simulink model "FPGA_Comm_test_plant"  (Simulink 7.6)
settings: Solver=ode4  StartTime=0.0  StopTime=500  FixedStep=0.01  MaxStep=1e-1  RelTol=1e-3
values from neighbouring files (symbols this model uses):
  s1 = op1(1)    [fpu_test.m]
settings Model: Creator=jordan  LastModifiedBy=jordan
settings GRTTargetCC: ExtMode=on

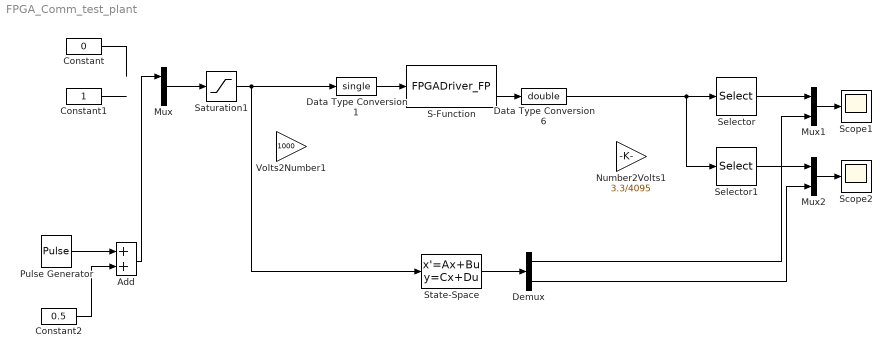
== system FPGA_Comm_test_plant ==
  Add : Sum
  Constant : Constant  Value=0
  Constant1 : Constant
  Constant2 : Constant  Value=0.5
  Data Type Conversion1 : DataTypeConversion  OutDataTypeStr=single
  Data Type Conversion6 : DataTypeConversion  OutDataTypeStr=double
  Demux : Demux  Outputs=2
  Mux : Mux  Inputs=2
  Mux1 : Mux  Inputs=2
  Mux2 : Mux  Inputs=2
  Number2Volts1 : Gain  Gain=3.3/4095
  Pulse Generator : DiscretePulseGenerator  PulseType=Time based  Period=10  PulseWidth=50
  S-Function : S-Function  FunctionName=FPGADriver_FP  EnableBusSupport=off
  Saturation1 : Saturate  UpperLimit=3  LowerLimit=0  LinearizeAsGain=off  RndMeth=Nearest
  Scope1 : Scope
      settings: TimeRange=50  YMin=-0.25  YMax=4  MaxDataPoints=50000
  Scope2 : Scope
      settings: TimeRange=50  YMin=0  YMax=3.5  MaxDataPoints=50000
  Selector : Selector  InputPortWidth=2  IndexOptions=Index vector (dialog)  Indices=1  OutputSizes=1
  Selector1 : Selector  InputPortWidth=2  IndexOptions=Index vector (dialog)  Indices=2  OutputSizes=1
  State-Space : StateSpace  A=s1.a  B=s1.b  C=s1.c  D=s1.d
  Volts2Number1 : Gain  Gain=1000
  wires:
  S-Function/2 -> Data Type Conversion6/1
  Data Type Conversion1/1 -> S-Function/1
  Data Type Conversion6/1 -> Selector/1, Selector1/1
  Mux/1 -> Saturation1/1
  Selector/1 -> Mux1/1
  Selector1/1 -> Mux2/1
  Saturation1/1 -> State-Space/1, Data Type Conversion1/1
  Mux1/1 -> Scope1/1
  Demux/1 -> Mux1/2
  State-Space/1 -> Demux/1
  Mux2/1 -> Scope2/1
  Demux/2 -> Mux2/2
  Pulse Generator/1 -> Add/1
  Constant2/1 -> Add/2
  Constant/1 -> ?
  Constant1/1 -> ?
  Add/1 -> Mux/1
